simulink model "continuo"  (R2019a)
settings: Solver=VariableStepAuto  StartTime=0.0  StopTime=20  RelTol=1e-3
libraries: simulink x1
settings Model: Creator=STEVEN  LastModifiedBy=STEVEN

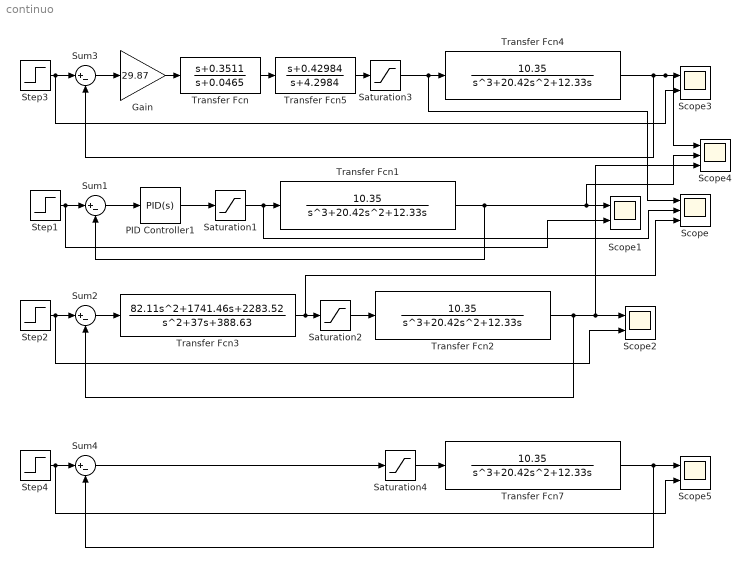
== system continuo ==
  Gain : Gain  Gain=29.87
  PID Controller1 : simulink/Continuous/PID Controller  Controller=PID  Form=Parallel  TimeDomain=Continuous-time  SampleTime=-1  IntegratorMethod=Forward Euler  FilterMethod=Forward Euler  ControllerParametersSource=internal  P=6.6771  I=0  D=4.5325  UseFilter=on  N=100  TunerSelectOption=Transfer Function Based (PID Tuner App)  InitialConditionSource=internal  InitialConditionForIntegrator=0  InitialConditionForFilter=0  DifferentiatorICPrevScaledInput=0  ExternalReset=none  TrackingMode=off  Kt=1  LimitOutput=off  UpperSaturationLimit=inf  LowerSaturationLimit=-inf  LinearizeAsGain=on  AntiWindupMode=none  Kb=1  POutMin=[]  POutMax=[]  IOutMin=[]  IOutMax=[]  DOutMin=[]  DOutMax=[]  NOutMin=[]  NOutMax=[]  SumOutMin=[]  SumOutMax=[]  SaturationOutMin=[]  SaturationOutMax=[]  PParamMin=[]  PParamMax=[]  IParamMin=[]  IParamMax=[]  DParamMin=[]  DParamMax=[]  NParamMin=[]  NParamMax=[]  KbParamMin=[]  KbParamMax=[]  KtParamMin=[]  KtParamMax=[]  KbOutMin=[]  KbOutMax=[]  KtOutMin=[]  KtOutMax=[]  IntegratorOutMin=[]  IntegratorOutMax=[]  FilterOutMin=[]  FilterOutMax=[]  SumI1OutMin=[]  SumI1OutMax=[]  SumI2OutMin=[]  SumI2OutMax=[]  SumI3OutMin=[]  SumI3OutMax=[]  SumI4OutMin=[]  SumI4OutMax=[]  SumDOutMin=[]  SumDOutMax=[]  DifferentiatorOutMin=[]  DifferentiatorOutMax=[]  FilterDiffOutCoefMin=[]  FilterDiffOutCoefMax=[]  ReciprocalOutMin=[]  ReciprocalOutMax=[]  SumDenOutMin=[]  SumDenOutMax=[]  SumNumOutMin=[]  SumNumOutMax=[]  DivideOutMin=[]  DivideOutMax=[]  IntegratorContinuousStateAttributes=''  IntegratorStateMustResolveToSignalObject=off  IntegratorRTWStateStorageClass=Auto  FilterContinuousStateAttributes=''  FilterStateMustResolveToSignalObject=off  FilterRTWStateStorageClass=Auto  ParallelPVariant=InternalParameters  IdealPVariant=Disabled  IVariant=InternalParameters  DVariant=InternalParameters  IntegratorVariant=Continuous  SatVariant=Disabled  AWVariant=Passthrough  PCopyVariant=Disabled  TRVariant=Disabled  FdbkBlocksVariant=Forward  IdealPFdbkVariant=Disabled  SatFdbkVariant=Disabled  DerivativeFilterVariant=ContFilter  NVariant=InternalParameters  NCopyVariant=Disabled  FilterICVariant=InternalICsFilter  IntegratorICVariant=InternalICs  ExternalResetVariant=Disabled  TRSumVariant=Passthrough  SumFdbkVariant=Disabled  SumVariant=Sum_PID
  Saturation{1..4} (4 alike) : Saturate  UpperLimit=10  LowerLimit=-10
  Scope : Scope  NumInputPorts=3
  Scope{1..3,5} (4 alike) : Scope  NumInputPorts=2
  Scope4 : Scope  NumInputPorts=3
  Step{1..4} (4 alike) : Step  Time=0  SampleTime=0
  Sum{1..4} (4 alike) : Sum  Inputs=|+-
  Transfer Fcn : TransferFcn  Numerator=[1 0.3511]  Denominator=[1 0.0465]
  Transfer Fcn{1..2,4,7} (4 alike) : TransferFcn  Numerator=10.35  Denominator=[1 20.42 12.33 0]
  Transfer Fcn3 : TransferFcn  Numerator=[82.11 1741.46 2283.52]  Denominator=[1 37 388.63]
  Transfer Fcn5 : TransferFcn  Numerator=[1 0.42984]  Denominator=[1 4.2984]
  wires:
  Step1/1 -> Scope1/2, Sum1/1
  Sum1/1 -> PID Controller1/1
  PID Controller1/1 -> Saturation1/1
  Saturation1/1 -> Scope/2, Transfer Fcn1/1
  Step2/1 -> Scope2/2, Sum2/1
  Transfer Fcn2/1 -> Sum2/2, Scope4/3, Scope2/1
  Sum2/1 -> Transfer Fcn3/1
  Transfer Fcn3/1 -> Scope/3, Saturation2/1
  Saturation2/1 -> Transfer Fcn2/1
  Step3/1 -> Scope3/2, Sum3/1
  Saturation3/1 -> Scope/1, Transfer Fcn4/1
  Sum3/1 -> Gain/1
  Transfer Fcn5/1 -> Saturation3/1
  Transfer Fcn4/1 -> Sum3/2, Scope4/1, Scope3/1
  Gain/1 -> Transfer Fcn/1
  Transfer Fcn/1 -> Transfer Fcn5/1
  Transfer Fcn1/1 -> Sum1/2, Scope4/2, Scope1/1
  Transfer Fcn7/1 -> Sum4/2, Scope5/1
  Step4/1 -> Scope5/2, Sum4/1
  Saturation4/1 -> Transfer Fcn7/1
  Sum4/1 -> Saturation4/1
